simulink model "Model_RLC_14b"  (R2014b)
settings: Solver=ode45  StartTime=0.0  StopTime=10.0  MaxStep=10-5  RelTol=1e-3
undefined symbols (not defined in the file or in its folder): in, param
libraries: simulink x1
settings Model: Creator=Zer0  LastModifiedBy=Arek

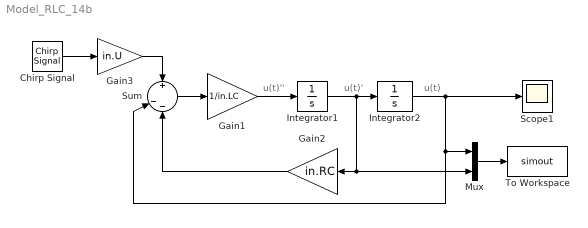
== system Model_RLC_14b ==
  note: u(t)
  note: u(t)'
  note: u(t)''
  Chirp Signal : simulink/Sources/Chirp Signal  f1=freq.fmin  T=param.tmax  f2=freq.fmax
  Gain1 : Gain  Gain=1/in.LC
  Gain2 : Gain  Gain=in.RC
  Gain3 : Gain  Gain=in.U
  Integrator1 : Integrator  InitialCondition=param.ic(2)
  Integrator2 : Integrator  InitialCondition=param.ic(1)
  Mux : Mux  Inputs=2
  Scope1 : Scope
      settings: YMin=-60  YMax=60
  Sum : Sum  Inputs=+|--
  To Workspace : ToWorkspace  VariableName=simout  SaveFormat=Timeseries  SampleTime=-1
  wires:
  Integrator1/1 -> Mux/2, Gain2/1, Integrator2/1
  Gain1/1 -> Integrator1/1
  Sum/1 -> Gain1/1
  Integrator2/1 -> Scope1/1, Mux/1, Sum/2
  Gain2/1 -> Sum/3
  Gain3/1 -> Sum/1
  Mux/1 -> To Workspace/1
  Chirp Signal/1 -> Gain3/1
